simulink model "mpc_control_constraints_N"  (R2023a)
settings: Solver=VariableStepAuto  StartTime=0.0  StopTime=0.5  RelTol=1e-3
values from neighbouring files (symbols this model uses):
  B_tilda = [sysdis.B(1) Bw_bar(1,1) Bw_bar(1,2); sysdis.B(2) Bw_bar(2,1) Bw_bar(2,2)]    [motor.m]
  D_tilda = [0 0 0 ; 0 0 0]    [motor.m]
  N1 = 5    [motor.m]
  N2 = 100    [motor.m]
  Q1 = Q_LQ    [motor.m]
  Q2 = Q_LQ    [motor.m]
  R1 = R_LQ    (= 1)    [motor.m]
  R2 = R_LQ    (= 1)    [motor.m]
  S1 = zeros(2)    [motor.m]
  S2 = zeros(2)    [motor.m]
  sysdis = c2d(sys,Ts)    [motor.m]
  Ts = 0.001    [parameters.m]
  u_max = 12    [constraints.m]
  u_min = 0    [constraints.m]
  uBar = -(A(1,1)*(-A(2,2)*nref/A(2,1)) + A(1,2)*nref)*L    [motor.m]
  w = [1 1]'    [parameters.m]
  x0 = [0.2 70.3]'    [motor.m]
  yref = [iref nref]'    [motor.m]
undefined symbols (not defined in the file or in its folder): motor_mpc
settings Model: Creator=teora  LastModifiedBy=teora

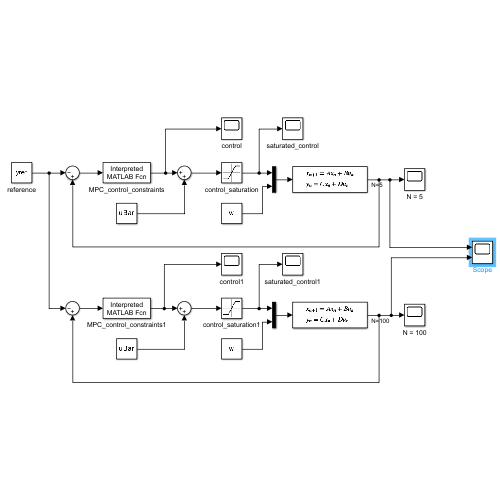
[thumbnail: Simulink's stored preview of the top-level diagram]
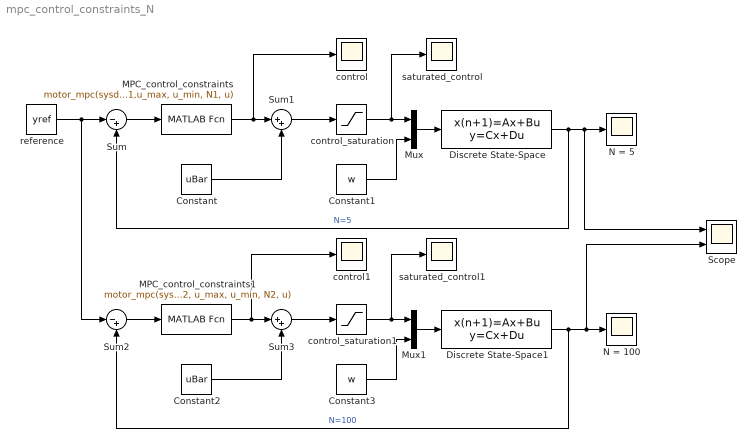
== system mpc_control_constraints_N ==
  Constant : Constant  Value=uBar
  Constant1 : Constant  Value=w
  Constant2 : Constant  Value=uBar
  Constant3 : Constant  Value=w
  Discrete State-Space : DiscreteStateSpace  A=sysdis.A  B=B_tilda  C=sysdis.C  D=D_tilda  InitialCondition=x0  SampleTime=Ts
  Discrete State-Space1 : DiscreteStateSpace  A=sysdis.A  B=B_tilda  C=sysdis.C  D=D_tilda  InitialCondition=x0  SampleTime=Ts
  MPC_control_constraints : MATLABFcn  MATLABFcn=motor_mpc(sysdis.A, sysdis.B, Q1, R1, S1,u_max, u_min, N1, u)  OutputDimensions=1
  MPC_control_constraints1 : MATLABFcn  MATLABFcn=motor_mpc(sysdis.A, sysdis.B, Q2, R2, S2, u_max, u_min, N2, u)  OutputDimensions=1
  Mux : Mux  Inputs=2
  Mux1 : Mux  Inputs=2
  N = 100 : Scope
  N = 5 : Scope
  Scope : Scope  NumInputPorts=2
  Sum : Sum  Inputs=|-+
  Sum1 : Sum  Inputs=|++
  Sum2 : Sum  Inputs=|-+
  Sum3 : Sum  Inputs=|++
  control : Scope
  control1 : Scope
  control_saturation : Saturate  UpperLimit=u_max  LowerLimit=u_min
  control_saturation1 : Saturate  UpperLimit=u_max  LowerLimit=u_min
  reference : Constant  Value=yref
  saturated_control : Scope
  saturated_control1 : Scope
  wires:
  Sum/1 -> MPC_control_constraints/1
  Discrete State-Space/1 -> Scope/1, N = 5/1, Sum/2  "N=5"
  Constant/1 -> Sum1/2
  control_saturation/1 -> saturated_control/1, Mux/1
  Mux/1 -> Discrete State-Space/1
  Constant1/1 -> Mux/2
  MPC_control_constraints/1 -> control/1, Sum1/1
  Sum1/1 -> control_saturation/1
  reference/1 -> Sum2/1, Sum/1
  Sum2/1 -> MPC_control_constraints1/1
  Discrete State-Space1/1 -> Scope/2, N = 100/1, Sum2/2  "N=100"
  Constant2/1 -> Sum3/2
  control_saturation1/1 -> saturated_control1/1, Mux1/1
  Mux1/1 -> Discrete State-Space1/1
  Constant3/1 -> Mux1/2
  MPC_control_constraints1/1 -> control1/1, Sum3/1
  Sum3/1 -> control_saturation1/1
